simulink model "discrete_intersample_ripple"  (R2021b)
settings: Solver=VariableStepAuto  StartTime=0.0  StopTime=10.0  RelTol=1e-3
libraries: cstblocks x2
settings Model: Creator=varunsampat  LastModifiedBy=varunsampat

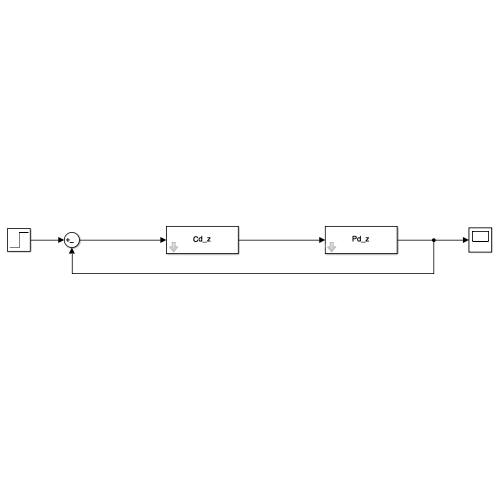
[thumbnail: Simulink's stored preview of the top-level diagram]
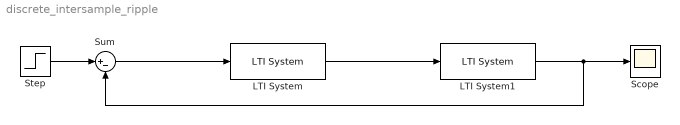
== system discrete_intersample_ripple ==
  LTI System : cstblocks/LTI System  sys=Cd_z  IC=[]
  LTI System1 : cstblocks/LTI System  sys=Pd_z  IC=[]
  Scope : Scope
  Step : Step  SampleTime=0
  Sum : Sum  Inputs=|+-
  wires:
  LTI System1/1 -> Sum/2, Scope/1
  Step/1 -> Sum/1
  Sum/1 -> LTI System/1
  LTI System/1 -> LTI System1/1
